simulink model "GlucodeModel"  (R2016a)
settings: Solver=VariableStepAuto  StartTime=0.0  StopTime=2000  RelTol=1e-3
libraries: simulink x1
settings Model: Creator=Dylan  LastModifiedBy=Dylan

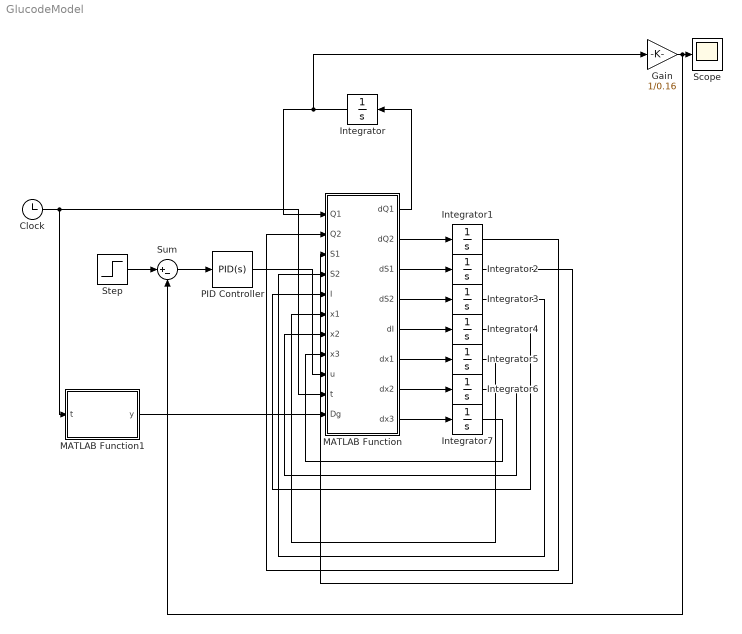
== system GlucodeModel ==
  Clock : Clock
  Gain : Gain  Gain=1/0.16
  Integrator : Integrator  InitialCondition=6*0.16
  Integrator{1..7} (7 alike) : Integrator
  MATLAB Function : MATLAB Function  TreatAsAtomicUnit=on
  MATLAB Function1 : MATLAB Function  TreatAsAtomicUnit=on
  PID Controller : simulink/Continuous/PID Controller  Controller=PID  TimeDomain=Continuous-time  SampleTime=-1  IntegratorMethod=Forward Euler  FilterMethod=Forward Euler  Form=Parallel  UseFilter=on  ControllerParametersSource=internal  P=0  I=0  D=0  N=0.41647001505876  InitialConditionSource=internal  InitialConditionForIntegrator=0  InitialConditionForFilter=0  ExternalReset=none  LimitOutput=off  UpperSaturationLimit=inf  LowerSaturationLimit=-inf  LinearizeAsGain=on  AntiWindupMode=none  Kb=1  TrackingMode=off  Kt=1  PParamMin=[]  PParamMax=[]  IParamMin=[]  IParamMax=[]  DParamMin=[]  DParamMax=[]  NParamMin=[]  NParamMax=[]  KbParamMin=[]  KbParamMax=[]  KtParamMin=[]  KtParamMax=[]  POutMin=[]  POutMax=[]  IOutMin=[]  IOutMax=[]  DOutMin=[]  DOutMax=[]  NOutMin=[]  NOutMax=[]  KbOutMin=[]  KbOutMax=[]  KtOutMin=[]  KtOutMax=[]  IntegratorOutMin=[]  IntegratorOutMax=[]  FilterOutMin=[]  FilterOutMax=[]  SumOutMin=[]  SumOutMax=[]  SumI1OutMin=[]  SumI1OutMax=[]  SumI2OutMin=[]  SumI2OutMax=[]  SumI3OutMin=[]  SumI3OutMax=[]  SumDOutMin=[]  SumDOutMax=[]  SaturationOutMin=[]  SaturationOutMax=[]  IntegratorContinuousStateAttributes=''  IntegratorStateMustResolveToSignalObject=off  IntegratorRTWStateStorageClass=Auto  FilterContinuousStateAttributes=''  FilterStateMustResolveToSignalObject=off  FilterRTWStateStorageClass=Auto  DifferentiatorICPrevScaledInput=0  DifferentiatorOutMin=[]  DifferentiatorOutMax=[]
  Scope : Scope
  Step : Step  Time=0  After=5  SampleTime=0
  Sum : Sum  Inputs=|+-
  wires:
  PID Controller/1 -> MATLAB Function/9(u)
  Sum/1 -> PID Controller/1
  Step/1 -> Sum/1
  Clock/1 -> MATLAB Function/10(t), MATLAB Function1/1(t)
  MATLAB Function/1(dQ1) -> Integrator/1
  MATLAB Function/8(dx3) -> Integrator7/1
  Integrator7/1 -> MATLAB Function/8(x3)
  MATLAB Function/2(dQ2) -> Integrator1/1
  MATLAB Function/3(dS1) -> Integrator2/1
  MATLAB Function/4(dS2) -> Integrator3/1
  MATLAB Function/5(dI) -> Integrator4/1
  MATLAB Function/6(dx1) -> Integrator5/1
  MATLAB Function/7(dx2) -> Integrator6/1
  Integrator6/1 -> MATLAB Function/7(x2)
  Integrator5/1 -> MATLAB Function/6(x1)
  Integrator4/1 -> MATLAB Function/5(I)
  Integrator3/1 -> MATLAB Function/4(S2)
  Integrator2/1 -> MATLAB Function/3(S1)
  Integrator1/1 -> MATLAB Function/2(Q2)
  MATLAB Function1/1(y) -> MATLAB Function/11(Dg)
  Gain/1 -> Sum/2, Scope/1
  Integrator/1 -> Gain/1, MATLAB Function/1(Q1)

== matlab function GlucodeModel/MATLAB Function1 ==
  data: t input; y output
function y = fcn(t)

y=1;

== matlab function GlucodeModel/MATLAB Function ==
  data: Q1 input; Q2 input; S1 input; S2 input; I input; x1 input; x2 input; x3 input; u input; t input; dQ1 output; dQ2 output; dS1 output; dS2 output; dI output; dx1 output; dx2 output; dx3 output; Dg input
function [dQ1, dQ2, dS1, dS2, dI, dx1, dx2, dx3]   = fcn(Q1, Q2, S1, S2, I, x1, x2, x3,u,t, Dg)
param = zeros(15,1);
param(1) = 0.066;
param(2) = 0.006;
param(3) = 0.06;
param(4) = 0.03;
param(5) = 0.138;
param(6) = 0.12;
param(7) = 0.16;
param(8) = 0.8;
param(9) = 40;
param(10) = 51.2*10^-4;
param(11) = 8.2*10^-4;
param(12) = 520*10^-4;
param(13) = 0.0161;
param(14) = 0.0097;
param(15) = 55;

x=zeros(8,1);
x(1) = Q1;
x(2) = Q2;
x(3) = S1;
x(4) = S2;
x(5) = I;
x(6) = x1;
x(7) = x2;
x(8) = x3;

    %Defining parameters
    k12 = param(1);
    ka1 = param(2);
    ka2 = param(3);
    ka3 = param(4);
    ke = param(5);
    VI = param(6);
    Vg = param(7);
    Ag = param(8);
    tmaxG = param(9);
    kb1 = param(10)*ka1;
    kb2 = param(11)*ka2;
    kb3 = param(12)*ka3;
    EGP0 = param(13);
    F01 = param(14);
    tmaxI = param(15);

%Formulized parameters
    G = x(1)/Vg;
    Ug = (Dg*Ag*t*exp(-t/tmaxG))/tmaxG^2;
    UI = x(4)/tmaxI;
    
    if G >= 4.5
        F01c = F01;
    else
        F01c = F01*G/4.5;
    end
    
    if G >= 9
        Fr = 0.003*(G-9)*Vg;
    else
        Fr = 0;
    end

    %System equations
    dQ1 = -(F01c/Vg*G+x(6))*x(1)+k12*x(2)-Fr+Ug+EGP0*(1-x(8)); %dQ1/dt
    dQ2 = x(6)*x(1)-(k12+x(7))*x(2); %dQ2/dt
    dS1 = u-x(3)/tmaxI; %dS1/dt;
    dS2 = x(3)/tmaxI - x(4)/tmaxI; %dS2/dt
    dI = UI/VI-ke*x(5);
    dx1 = -ka1*x(6)+kb1*x(5);
    dx2 = -ka2*x(7)+kb2*x(5);
    dx3 = -ka3*x(8)+kb3*x(5);    %Formulized parameters
    G = x(1)/Vg;
    Ug = (Dg*Ag*t*exp(-t/tmaxG))/tmaxG^2;
    UI = x(4)/tmaxI;
    
    if G >= 4.5
        F01c = F01;
    else
        F01c = F01*G/4.5;
    end
    
    if G >= 9
        Fr = 0.003*(G-9)*Vg;
    else
        Fr = 0;
    end

    %System equations
    xdot=zeros(8,1);
    xdot(1) = -(F01c/(Vg*G)+x(6))*x(1)+k12*x(2)-Fr+Ug+EGP0*(1-x(8)); %dQ1/dt
    xdot(2) = x(6)*x(1)-(k12+x(7))*x(2); %dQ2/dt
    xdot(3) = u-x(3)/tmaxI; %dS1/dt;
    xdot(4) = x(3)/tmaxI - x(4)/tmaxI; %dS2/dt
    xdot(5) = UI/VI-ke*x(5);
    xdot(6) = -ka1*x(6)+kb1*x(5);
    xdot(7) = -ka2*x(7)+kb2*x(5);
    xdot(8) = -ka3*x(8)+kb3*x(5);

end
